simulink model "Ext_MFTyre_MFSwift_2sf"  (R2016b)
settings: Solver=ode4  StartTime=0.0  StopTime=20  FixedStep=0.0005  RelTol=1e-3
libraries: simulink_extras x16, mfswift_library x4, Solver_SF x2
settings Model: Creator=ywata  LastModifiedBy=mkhan
settings SolverCC: AutoInsertRateTranBlk=on
settings DataIOCC: ReturnWorkspaceOutputs=on
settings OptimizationCC: LifeSpan=inf
settings SFSimCC: SimUseLocalCustomCode=on
settings RTWCC: RTWUseLocalCustomCode=on

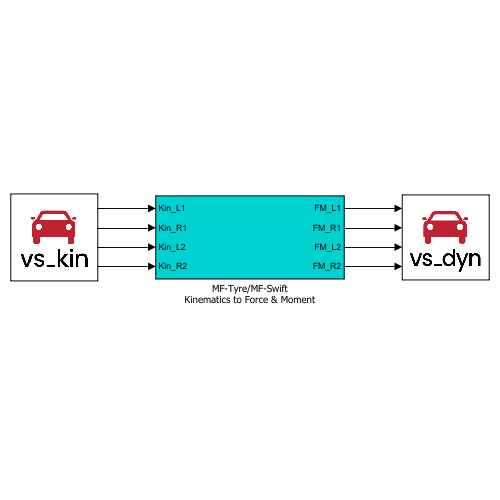
[thumbnail: Simulink's stored preview of the top-level diagram]
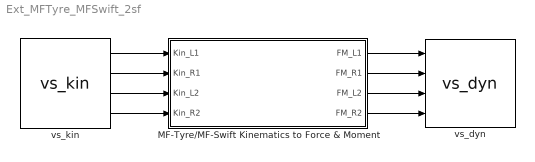
== system Ext_MFTyre_MFSwift_2sf ==
  MF-Tyre/MF-Swift Kinematics to Force & Moment : Subsystem
  vs_dyn : Solver_SF/CarSim Multi-Wrappers/vs_dyn  Priority=4  SIMFILE=simfile.sim
  vs_kin : Solver_SF/CarSim Multi-Wrappers/vs_kin  Priority=3  SIMFILE=simfile.sim
  wires:
  vs_kin/3 -> MF-Tyre/MF-Swift Kinematics to Force & Moment/3(Kin_L2)
  vs_kin/1 -> MF-Tyre/MF-Swift Kinematics to Force & Moment/1(Kin_L1)
  MF-Tyre/MF-Swift Kinematics to Force & Moment/1(FM_L1) -> vs_dyn/1
  MF-Tyre/MF-Swift Kinematics to Force & Moment/3(FM_L2) -> vs_dyn/3
  MF-Tyre/MF-Swift Kinematics to Force & Moment/2(FM_R1) -> vs_dyn/2
  MF-Tyre/MF-Swift Kinematics to Force & Moment/4(FM_R2) -> vs_dyn/4
  vs_kin/2 -> MF-Tyre/MF-Swift Kinematics to Force & Moment/2(Kin_R1)
  vs_kin/4 -> MF-Tyre/MF-Swift Kinematics to Force & Moment/4(Kin_R2)

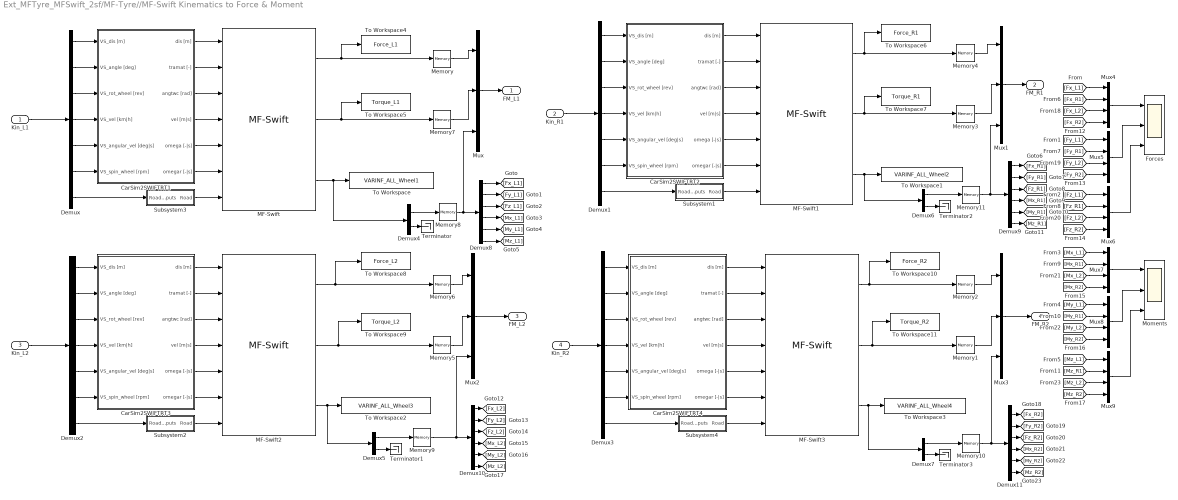
== system Ext_MFTyre_MFSwift_2sf/MF-Tyre//MF-Swift Kinematics to Force & Moment ==
  Kin_L1 : Inport
  Kin_R1 : Inport  Port=2
  Kin_L2 : Inport  Port=3
  Kin_R2 : Inport  Port=4
  CarSim2SWIFTRT1 : Subsystem
  CarSim2SWIFTRT2 : Subsystem
  CarSim2SWIFTRT3 : Subsystem
  CarSim2SWIFTRT4 : Subsystem
  Demux{,1..3} (4 alike) : Demux  Outputs=[3 3 1 3 3 1 3]
  Demux{8..11} (4 alike) : Demux  Outputs=6
  Demux4 : Demux  Outputs=[6 54]
  Demux5 : Demux  Outputs=[6 54]
  Demux6 : Demux  Outputs=[6,54]
  Demux7 : Demux  Outputs=[6 54]
  Forces : Scope  NumInputPorts=3
  MF-Swift : mfswift_library/MF-Swift  idtyre=1  tpfname='CS_car225_60R18.tir'  rdfname=''  road_mode=(3xxxx) external  side_mode=(x3xxx) symmetric  cnt_mode=(xx1xx) smooth road  dyn_mode=(xxx1x) relaxation behaviour  mf_mode=(xxxx4) combined  tv_model=Disabled  overwrite=off  use_mode=1e8  internal_solver=off  enable_rr_init=on  disp_debug=off
  MF-Swift1 : mfswift_library/MF-Swift  idtyre=2  tpfname='CS_car225_60R18.tir'  rdfname=''  road_mode=(3xxxx) external  side_mode=(x3xxx) symmetric  cnt_mode=(xx1xx) smooth road  dyn_mode=(xxx1x) relaxation behaviour  mf_mode=(xxxx4) combined  tv_model=Disabled  overwrite=off  use_mode=1e8  internal_solver=off  enable_rr_init=on  disp_debug=off
  MF-Swift2 : mfswift_library/MF-Swift  idtyre=3  tpfname='CS_car225_60R18.tir'  rdfname=''  road_mode=(3xxxx) external  side_mode=(x3xxx) symmetric  cnt_mode=(xx1xx) smooth road  dyn_mode=(xxx1x) relaxation behaviour  mf_mode=(xxxx4) combined  tv_model=Disabled  overwrite=off  use_mode=1e8  internal_solver=off  enable_rr_init=on  disp_debug=off
  MF-Swift3 : mfswift_library/MF-Swift  idtyre=4  tpfname='CS_car225_60R18.tir'  rdfname=''  road_mode=(3xxxx) external  side_mode=(x3xxx) symmetric  cnt_mode=(xx1xx) smooth road  dyn_mode=(xxx1x) relaxation behaviour  mf_mode=(xxxx4) combined  tv_model=Disabled  overwrite=off  use_mode=1e8  internal_solver=off  enable_rr_init=on  disp_debug=off
  Memory{,1..11} (12 alike) : Memory
  Moments : Scope  NumInputPorts=3
  Mux{,1..3} (4 alike) : Mux  Inputs=[3 3 6]
  Mux{4..9} (6 alike) : Mux
  Subsystem1 : Subsystem
  Subsystem2 : Subsystem
  Subsystem3 : Subsystem
  Subsystem4 : Subsystem
  Terminator{,1..3} (4 alike) : Terminator
  To Workspace : ToWorkspace  VariableName=VARINF_ALL_Wheel1  SampleTime=-1
  To Workspace1 : ToWorkspace  VariableName=VARINF_ALL_Wheel2  SampleTime=-1
  To Workspace10 : ToWorkspace  VariableName=Force_R2  SampleTime=-1
  To Workspace11 : ToWorkspace  VariableName=Torque_R2  SampleTime=-1
  To Workspace2 : ToWorkspace  VariableName=VARINF_ALL_Wheel3  SampleTime=-1
  To Workspace3 : ToWorkspace  VariableName=VARINF_ALL_Wheel4  SampleTime=-1
  To Workspace4 : ToWorkspace  VariableName=Force_L1  SampleTime=-1
  To Workspace5 : ToWorkspace  VariableName=Torque_L1  SampleTime=-1
  To Workspace6 : ToWorkspace  VariableName=Force_R1  SampleTime=-1
  To Workspace7 : ToWorkspace  VariableName=Torque_R1  SampleTime=-1
  To Workspace8 : ToWorkspace  VariableName=Force_L2  SampleTime=-1
  To Workspace9 : ToWorkspace  VariableName=Torque_L2  SampleTime=-1
  FM_L1 : Outport
  FM_R1 : Outport  Port=2
  FM_L2 : Outport  Port=3
  FM_R2 : Outport  Port=4
  wires:
  Mux/1 -> FM_L1/1
  Kin_L1/1 -> Demux/1
  MF-Swift1/1 -> Memory4/1, To Workspace6/1
  MF-Swift1/3 -> Demux6/1, To Workspace1/1
  CarSim2SWIFTRT2/1(dis [m]) -> MF-Swift1/1
  CarSim2SWIFTRT2/2(tramat [-]) -> MF-Swift1/2
  CarSim2SWIFTRT2/4(vel [m|s]) -> MF-Swift1/4
  CarSim2SWIFTRT2/5(omega [-|s]) -> MF-Swift1/5
  CarSim2SWIFTRT2/6(omegar [-|s]) -> MF-Swift1/6
  Mux1/1 -> FM_R1/1
  CarSim2SWIFTRT2/3(angtwc [rad]) -> MF-Swift1/3
  MF-Swift2/3 -> Demux5/1, To Workspace2/1
  CarSim2SWIFTRT3/1(dis [m]) -> MF-Swift2/1
  CarSim2SWIFTRT3/2(tramat [-]) -> MF-Swift2/2
  CarSim2SWIFTRT3/3(angtwc [rad]) -> MF-Swift2/3
  CarSim2SWIFTRT3/4(vel [m|s]) -> MF-Swift2/4
  CarSim2SWIFTRT3/5(omega [-|s]) -> MF-Swift2/5
  CarSim2SWIFTRT3/6(omegar [-|s]) -> MF-Swift2/6
  Mux2/1 -> FM_L2/1
  MF-Swift3/3 -> Demux7/1, To Workspace3/1
  CarSim2SWIFTRT4/1(dis [m]) -> MF-Swift3/1
  CarSim2SWIFTRT4/2(tramat [-]) -> MF-Swift3/2
  CarSim2SWIFTRT4/3(angtwc [rad]) -> MF-Swift3/3
  CarSim2SWIFTRT4/4(vel [m|s]) -> MF-Swift3/4
  CarSim2SWIFTRT4/5(omega [-|s]) -> MF-Swift3/5
  CarSim2SWIFTRT4/6(omegar [-|s]) -> MF-Swift3/6
  Mux3/1 -> FM_R2/1
  MF-Swift/2 -> Memory7/1, To Workspace5/1
  MF-Swift2/2 -> Memory5/1, To Workspace9/1
  MF-Swift1/2 -> Memory3/1, To Workspace7/1
  MF-Swift3/2 -> Memory1/1, To Workspace11/1
  MF-Swift/1 -> Memory/1, To Workspace4/1
  MF-Swift2/1 -> Memory6/1, To Workspace8/1
  MF-Swift3/1 -> Memory2/1, To Workspace10/1
  Subsystem2/1(Road) -> MF-Swift2/7
  Subsystem1/1(Road) -> MF-Swift1/7
  Subsystem4/1(Road) -> MF-Swift3/7
  MF-Swift/3 -> Demux4/1, To Workspace/1
  CarSim2SWIFTRT1/1(dis [m]) -> MF-Swift/1
  CarSim2SWIFTRT1/2(tramat [-]) -> MF-Swift/2
  CarSim2SWIFTRT1/3(angtwc [rad]) -> MF-Swift/3
  CarSim2SWIFTRT1/4(vel [m|s]) -> MF-Swift/4
  CarSim2SWIFTRT1/5(omega [-|s]) -> MF-Swift/5
  CarSim2SWIFTRT1/6(omegar [-|s]) -> MF-Swift/6
  Subsystem3/1(Road) -> MF-Swift/7
  Memory/1 -> Mux/1
  Memory7/1 -> Mux/2
  Memory6/1 -> Mux2/1
  Memory5/1 -> Mux2/2
  Memory4/1 -> Mux1/1
  Memory3/1 -> Mux1/2
  Memory2/1 -> Mux3/1
  Memory1/1 -> Mux3/2
  Demux4/1 -> Memory8/1
  Memory8/1 -> Demux8/1, Mux/3
  Demux5/1 -> Memory9/1
  Demux7/1 -> Memory10/1
  Demux6/1 -> Memory11/1
  Demux4/2 -> Terminator/1
  Demux5/2 -> Terminator1/1
  Demux6/2 -> Terminator2/1
  Demux7/2 -> Terminator3/1
  Demux/6 -> CarSim2SWIFTRT1/6(VS_spin_wheel [rpm])
  Demux/5 -> CarSim2SWIFTRT1/5(VS_angular_vel [deg|s])
  Demux/4 -> CarSim2SWIFTRT1/4(VS_vel [km|h])
  Demux/3 -> CarSim2SWIFTRT1/3(VS_rot_wheel [rev])
  Demux/2 -> CarSim2SWIFTRT1/2(VS_angle [deg])
  Demux/1 -> CarSim2SWIFTRT1/1(VS_dis [m])
  Kin_L2/1 -> Demux2/1
  Demux2/6 -> CarSim2SWIFTRT3/6(VS_spin_wheel [rpm])
  Demux2/3 -> CarSim2SWIFTRT3/3(VS_rot_wheel [rev])
  Demux2/1 -> CarSim2SWIFTRT3/1(VS_dis [m])
  Demux2/2 -> CarSim2SWIFTRT3/2(VS_angle [deg])
  Demux2/5 -> CarSim2SWIFTRT3/5(VS_angular_vel [deg|s])
  Demux2/4 -> CarSim2SWIFTRT3/4(VS_vel [km|h])
  Kin_R1/1 -> Demux1/1
  Demux1/6 -> CarSim2SWIFTRT2/6(VS_spin_wheel [rpm])
  Demux1/3 -> CarSim2SWIFTRT2/3(VS_rot_wheel [rev])
  Demux1/1 -> CarSim2SWIFTRT2/1(VS_dis [m])
  Demux1/2 -> CarSim2SWIFTRT2/2(VS_angle [deg])
  Demux1/5 -> CarSim2SWIFTRT2/5(VS_angular_vel [deg|s])
  Demux1/4 -> CarSim2SWIFTRT2/4(VS_vel [km|h])
  Kin_R2/1 -> Demux3/1
  Demux3/6 -> CarSim2SWIFTRT4/6(VS_spin_wheel [rpm])
  Demux3/3 -> CarSim2SWIFTRT4/3(VS_rot_wheel [rev])
  Demux3/1 -> CarSim2SWIFTRT4/1(VS_dis [m])
  Demux3/2 -> CarSim2SWIFTRT4/2(VS_angle [deg])
  Demux3/5 -> CarSim2SWIFTRT4/5(VS_angular_vel [deg|s])
  Demux3/4 -> CarSim2SWIFTRT4/4(VS_vel [km|h])
  Demux8/1 -> [Fx_L1]
  Demux8/2 -> [Fy_L1]
  Demux8/3 -> [Fz_L1]
  Demux8/4 -> [Mx_L1]
  Demux8/5 -> [My_L1]
  Demux8/6 -> [Mz_L1]
  Memory11/1 -> Demux9/1, Mux1/3
  Demux9/1 -> [Fx_R1]
  Demux9/6 -> [Mz_R1]
  Demux9/4 -> [Mx_R1]
  Demux9/3 -> [Fz_R1]
  Demux9/5 -> [My_R1]
  Demux9/2 -> [Fy_R1]
  Memory9/1 -> Mux2/3, Demux10/1
  Demux10/1 -> [Fx_L2]
  Demux10/6 -> [Mz_L2]
  Demux10/4 -> [Mx_L2]
  Demux10/3 -> [Fz_L2]
  Demux10/5 -> [My_L2]
  Demux10/2 -> [Fy_L2]
  Memory10/1 -> Mux3/3, Demux11/1
  Demux11/1 -> [Fx_R2]
  Demux11/6 -> [Mz_R2]
  Demux11/4 -> [Mx_R2]
  Demux11/3 -> [Fz_R2]
  Demux11/5 -> [My_R2]
  Demux11/2 -> [Fy_R2]
  [Fx_L1] -> Mux4/1
  [Fx_L2] -> Mux4/3
  [Fx_R1] -> Mux4/2
  [Fx_R2] -> Mux4/4
  [Fy_L1] -> Mux5/1
  [Fy_R1] -> Mux5/2
  [Fy_L2] -> Mux5/3
  [Fy_R2] -> Mux5/4
  [Fz_L1] -> Mux6/1
  [Fz_R1] -> Mux6/2
  [Fz_L2] -> Mux6/3
  [Fz_R2] -> Mux6/4
  Mux4/1 -> Forces/1
  Mux5/1 -> Forces/2
  Mux6/1 -> Forces/3
  Mux9/1 -> Moments/3
  [My_R1] -> Mux8/2
  [Mx_L1] -> Mux7/1
  [My_R2] -> Mux8/4
  Mux8/1 -> Moments/2
  Mux7/1 -> Moments/1
  [Mx_L2] -> Mux7/3
  [My_L1] -> Mux8/1
  [Mz_R1] -> Mux9/2
  [Mx_R1] -> Mux7/2
  [Mx_R2] -> Mux7/4
  [Mz_R2] -> Mux9/4
  [My_L2] -> Mux8/3
  [Mz_L2] -> Mux9/3
  [Mz_L1] -> Mux9/1
  Demux/7 -> Subsystem3/1(Road imputs)
  Demux3/7 -> Subsystem4/1(Road imputs)
  Demux1/7 -> Subsystem1/1(Road imputs)
  Demux2/7 -> Subsystem2/1(Road imputs)

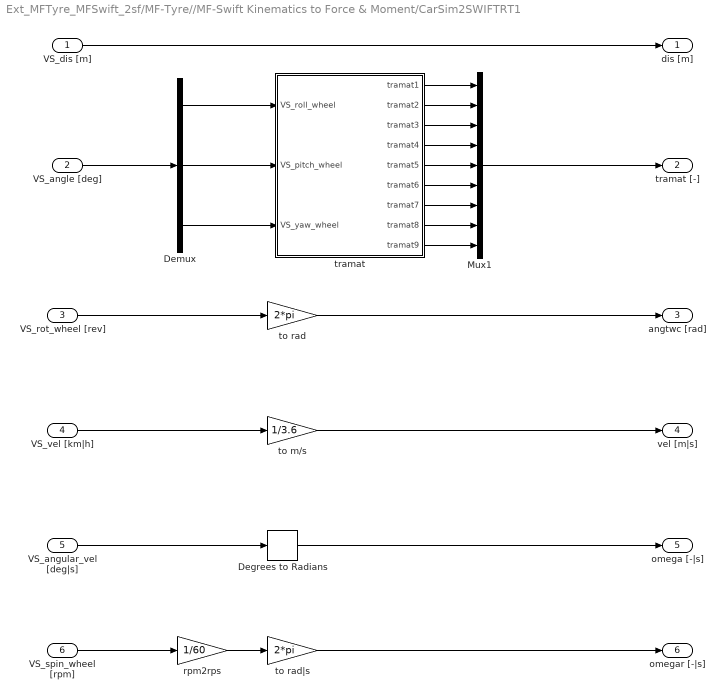
== system Ext_MFTyre_MFSwift_2sf/MF-Tyre//MF-Swift Kinematics to Force & Moment/CarSim2SWIFTRT1 ==
  VS_dis [m] : Inport
  VS_angle [deg] : Inport  Port=2
  VS_rot_wheel [rev] : Inport  Port=3
  VS_vel [km|h] : Inport  Port=4
  VS_angular_vel [deg|s] : Inport  Port=5
  VS_spin_wheel [rpm] : Inport  Port=6
  Degrees to Radians : simulink_extras/Transformations/Degrees to Radians
  Demux : Demux  Outputs=3
  Mux1 : Mux  Inputs=9
  rpm2rps : Gain  Gain=1/60
  to m/s : Gain  Gain=1/3.6
  to rad : Gain  Gain=2*pi
  to rad|s : Gain  Gain=2*pi
  tramat : Subsystem
  dis [m] : Outport
  tramat [-] : Outport  Port=2
  angtwc [rad] : Outport  Port=3
  vel [m|s] : Outport  Port=4
  omega [-|s] : Outport  Port=5
  omegar [-|s] : Outport  Port=6
  wires:
  Degrees to Radians/1 -> omega [-|s]/1
  to rad/1 -> angtwc [rad]/1
  tramat/1(tramat1) -> Mux1/1
  tramat/2(tramat2) -> Mux1/2
  tramat/3(tramat3) -> Mux1/3
  tramat/4(tramat4) -> Mux1/4
  tramat/5(tramat5) -> Mux1/5
  tramat/6(tramat6) -> Mux1/6
  tramat/7(tramat7) -> Mux1/7
  tramat/8(tramat8) -> Mux1/8
  tramat/9(tramat9) -> Mux1/9
  Mux1/1 -> tramat [-]/1
  VS_rot_wheel [rev]/1 -> to rad/1
  to m/s/1 -> vel [m|s]/1
  rpm2rps/1 -> to rad|s/1
  VS_spin_wheel [rpm]/1 -> rpm2rps/1
  to rad|s/1 -> omegar [-|s]/1
  VS_dis [m]/1 -> dis [m]/1
  VS_angle [deg]/1 -> Demux/1
  Demux/2 -> tramat/2(VS_pitch_wheel)
  Demux/1 -> tramat/1(VS_roll_wheel)
  Demux/3 -> tramat/3(VS_yaw_wheel)
  VS_vel [km|h]/1 -> to m/s/1
  VS_angular_vel [deg|s]/1 -> Degrees to Radians/1

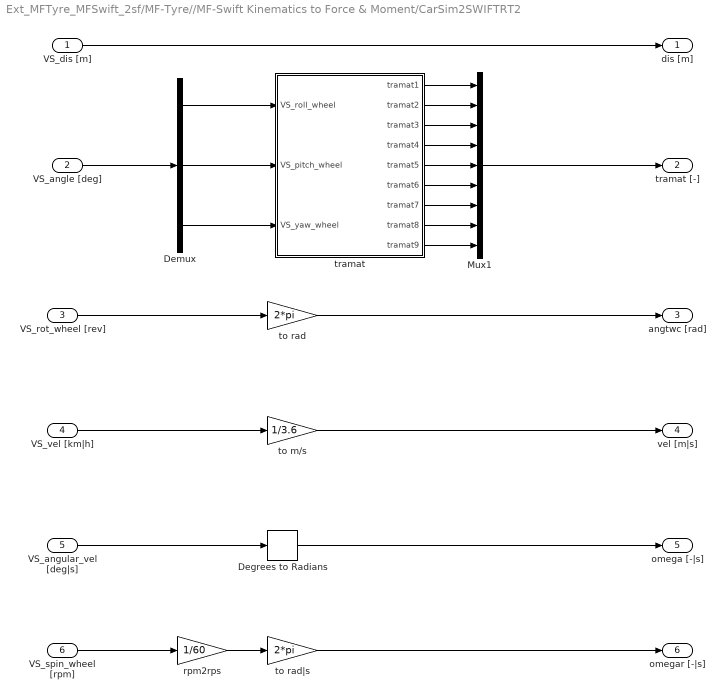
== system Ext_MFTyre_MFSwift_2sf/MF-Tyre//MF-Swift Kinematics to Force & Moment/CarSim2SWIFTRT2 ==
  VS_dis [m] : Inport
  VS_angle [deg] : Inport  Port=2
  VS_rot_wheel [rev] : Inport  Port=3
  VS_vel [km|h] : Inport  Port=4
  VS_angular_vel [deg|s] : Inport  Port=5
  VS_spin_wheel [rpm] : Inport  Port=6
  Degrees to Radians : simulink_extras/Transformations/Degrees to Radians
  Demux : Demux  Outputs=3
  Mux1 : Mux  Inputs=9
  rpm2rps : Gain  Gain=1/60
  to m/s : Gain  Gain=1/3.6
  to rad : Gain  Gain=2*pi
  to rad|s : Gain  Gain=2*pi
  tramat : Subsystem
  dis [m] : Outport
  tramat [-] : Outport  Port=2
  angtwc [rad] : Outport  Port=3
  vel [m|s] : Outport  Port=4
  omega [-|s] : Outport  Port=5
  omegar [-|s] : Outport  Port=6
  wires:
  Degrees to Radians/1 -> omega [-|s]/1
  to rad/1 -> angtwc [rad]/1
  tramat/1(tramat1) -> Mux1/1
  tramat/2(tramat2) -> Mux1/2
  tramat/3(tramat3) -> Mux1/3
  tramat/4(tramat4) -> Mux1/4
  tramat/5(tramat5) -> Mux1/5
  tramat/6(tramat6) -> Mux1/6
  tramat/7(tramat7) -> Mux1/7
  tramat/8(tramat8) -> Mux1/8
  tramat/9(tramat9) -> Mux1/9
  Mux1/1 -> tramat [-]/1
  VS_rot_wheel [rev]/1 -> to rad/1
  to m/s/1 -> vel [m|s]/1
  rpm2rps/1 -> to rad|s/1
  VS_spin_wheel [rpm]/1 -> rpm2rps/1
  to rad|s/1 -> omegar [-|s]/1
  VS_dis [m]/1 -> dis [m]/1
  VS_angle [deg]/1 -> Demux/1
  Demux/2 -> tramat/2(VS_pitch_wheel)
  Demux/1 -> tramat/1(VS_roll_wheel)
  Demux/3 -> tramat/3(VS_yaw_wheel)
  VS_vel [km|h]/1 -> to m/s/1
  VS_angular_vel [deg|s]/1 -> Degrees to Radians/1

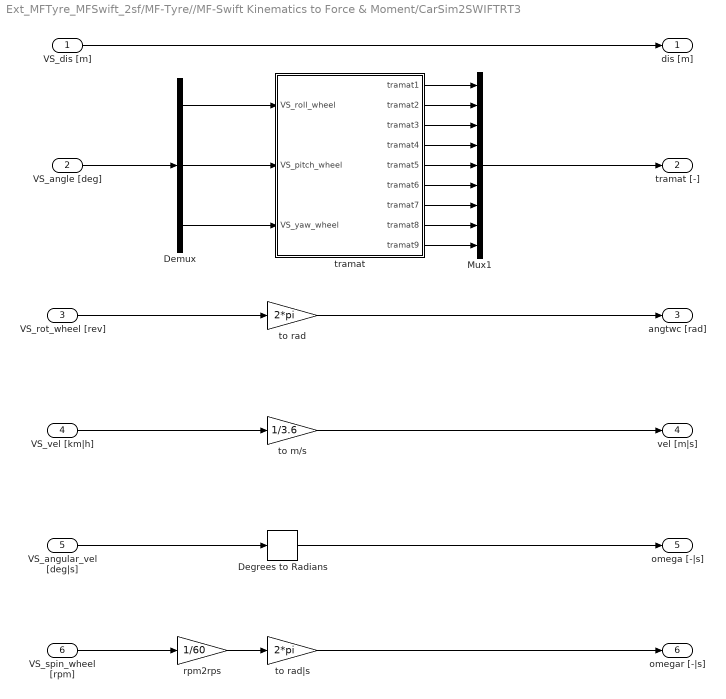
== system Ext_MFTyre_MFSwift_2sf/MF-Tyre//MF-Swift Kinematics to Force & Moment/CarSim2SWIFTRT3 ==
  VS_dis [m] : Inport
  VS_angle [deg] : Inport  Port=2
  VS_rot_wheel [rev] : Inport  Port=3
  VS_vel [km|h] : Inport  Port=4
  VS_angular_vel [deg|s] : Inport  Port=5
  VS_spin_wheel [rpm] : Inport  Port=6
  Degrees to Radians : simulink_extras/Transformations/Degrees to Radians
  Demux : Demux  Outputs=3
  Mux1 : Mux  Inputs=9
  rpm2rps : Gain  Gain=1/60
  to m/s : Gain  Gain=1/3.6
  to rad : Gain  Gain=2*pi
  to rad|s : Gain  Gain=2*pi
  tramat : Subsystem
  dis [m] : Outport
  tramat [-] : Outport  Port=2
  angtwc [rad] : Outport  Port=3
  vel [m|s] : Outport  Port=4
  omega [-|s] : Outport  Port=5
  omegar [-|s] : Outport  Port=6
  wires:
  Degrees to Radians/1 -> omega [-|s]/1
  to rad/1 -> angtwc [rad]/1
  tramat/1(tramat1) -> Mux1/1
  tramat/2(tramat2) -> Mux1/2
  tramat/3(tramat3) -> Mux1/3
  tramat/4(tramat4) -> Mux1/4
  tramat/5(tramat5) -> Mux1/5
  tramat/6(tramat6) -> Mux1/6
  tramat/7(tramat7) -> Mux1/7
  tramat/8(tramat8) -> Mux1/8
  tramat/9(tramat9) -> Mux1/9
  Mux1/1 -> tramat [-]/1
  VS_rot_wheel [rev]/1 -> to rad/1
  to m/s/1 -> vel [m|s]/1
  rpm2rps/1 -> to rad|s/1
  VS_spin_wheel [rpm]/1 -> rpm2rps/1
  to rad|s/1 -> omegar [-|s]/1
  VS_dis [m]/1 -> dis [m]/1
  VS_angle [deg]/1 -> Demux/1
  Demux/2 -> tramat/2(VS_pitch_wheel)
  Demux/1 -> tramat/1(VS_roll_wheel)
  Demux/3 -> tramat/3(VS_yaw_wheel)
  VS_vel [km|h]/1 -> to m/s/1
  VS_angular_vel [deg|s]/1 -> Degrees to Radians/1

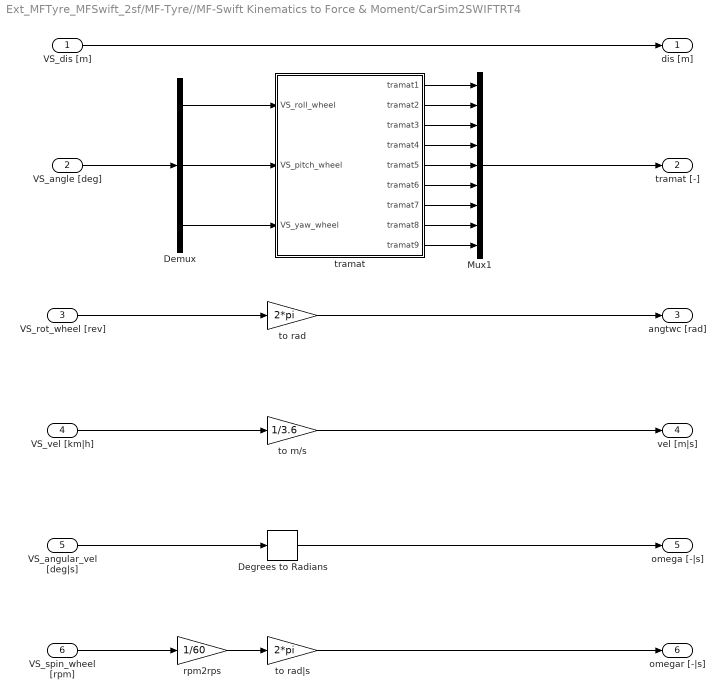
== system Ext_MFTyre_MFSwift_2sf/MF-Tyre//MF-Swift Kinematics to Force & Moment/CarSim2SWIFTRT4 ==
  VS_dis [m] : Inport
  VS_angle [deg] : Inport  Port=2
  VS_rot_wheel [rev] : Inport  Port=3
  VS_vel [km|h] : Inport  Port=4
  VS_angular_vel [deg|s] : Inport  Port=5
  VS_spin_wheel [rpm] : Inport  Port=6
  Degrees to Radians : simulink_extras/Transformations/Degrees to Radians
  Demux : Demux  Outputs=3
  Mux1 : Mux  Inputs=9
  rpm2rps : Gain  Gain=1/60
  to m/s : Gain  Gain=1/3.6
  to rad : Gain  Gain=2*pi
  to rad|s : Gain  Gain=2*pi
  tramat : Subsystem
  dis [m] : Outport
  tramat [-] : Outport  Port=2
  angtwc [rad] : Outport  Port=3
  vel [m|s] : Outport  Port=4
  omega [-|s] : Outport  Port=5
  omegar [-|s] : Outport  Port=6
  wires:
  Degrees to Radians/1 -> omega [-|s]/1
  to rad/1 -> angtwc [rad]/1
  tramat/1(tramat1) -> Mux1/1
  tramat/2(tramat2) -> Mux1/2
  tramat/3(tramat3) -> Mux1/3
  tramat/4(tramat4) -> Mux1/4
  tramat/5(tramat5) -> Mux1/5
  tramat/6(tramat6) -> Mux1/6
  tramat/7(tramat7) -> Mux1/7
  tramat/8(tramat8) -> Mux1/8
  tramat/9(tramat9) -> Mux1/9
  Mux1/1 -> tramat [-]/1
  VS_rot_wheel [rev]/1 -> to rad/1
  to m/s/1 -> vel [m|s]/1
  rpm2rps/1 -> to rad|s/1
  VS_spin_wheel [rpm]/1 -> rpm2rps/1
  to rad|s/1 -> omegar [-|s]/1
  VS_dis [m]/1 -> dis [m]/1
  VS_angle [deg]/1 -> Demux/1
  Demux/2 -> tramat/2(VS_pitch_wheel)
  Demux/1 -> tramat/1(VS_roll_wheel)
  Demux/3 -> tramat/3(VS_yaw_wheel)
  VS_vel [km|h]/1 -> to m/s/1
  VS_angular_vel [deg|s]/1 -> Degrees to Radians/1

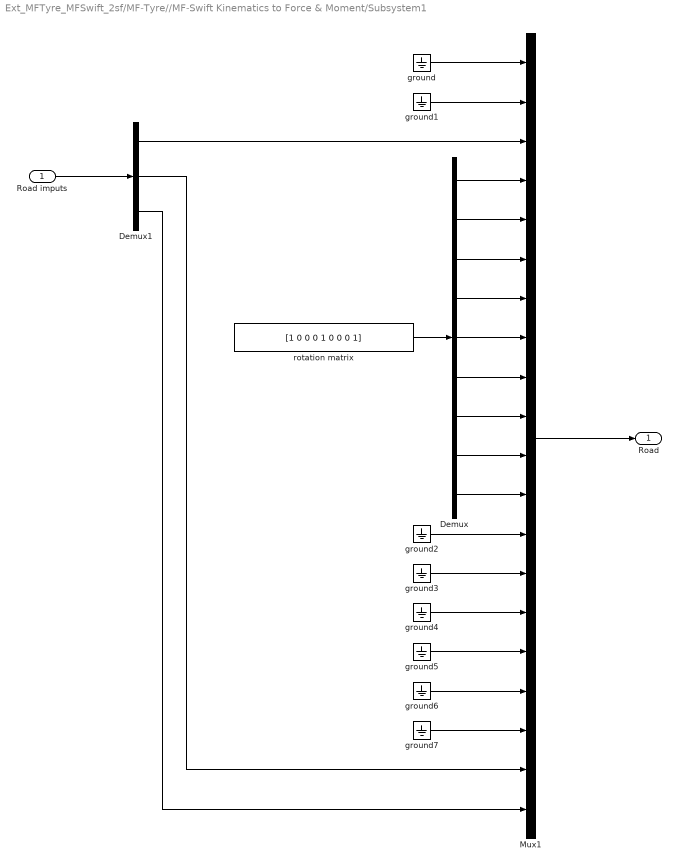
== system Ext_MFTyre_MFSwift_2sf/MF-Tyre//MF-Swift Kinematics to Force & Moment/Subsystem1 ==
  Road imputs : Inport
  Demux : Demux  Outputs=9
  Demux1 : Demux  Outputs=3
  Mux1 : Mux  Inputs=20
  ground{,1..7} (8 alike) : Ground
  rotation matrix : Constant  Value=[1 0 0 0 1 0 0 0 1]
  Road : Outport
  wires:
  Mux1/1 -> Road/1
  ground/1 -> Mux1/1
  ground1/1 -> Mux1/2
  ground2/1 -> Mux1/13
  ground3/1 -> Mux1/14
  ground4/1 -> Mux1/15
  ground5/1 -> Mux1/16
  ground6/1 -> Mux1/17
  ground7/1 -> Mux1/18
  Demux1/2 -> Mux1/19
  Demux1/3 -> Mux1/20
  rotation matrix/1 -> Demux/1
  Demux/1 -> Mux1/4
  Demux/2 -> Mux1/5
  Demux/3 -> Mux1/6
  Demux/4 -> Mux1/7
  Demux/5 -> Mux1/8
  Demux/6 -> Mux1/9
  Demux/7 -> Mux1/10
  Demux/8 -> Mux1/11
  Demux/9 -> Mux1/12
  Road imputs/1 -> Demux1/1
  Demux1/1 -> Mux1/3

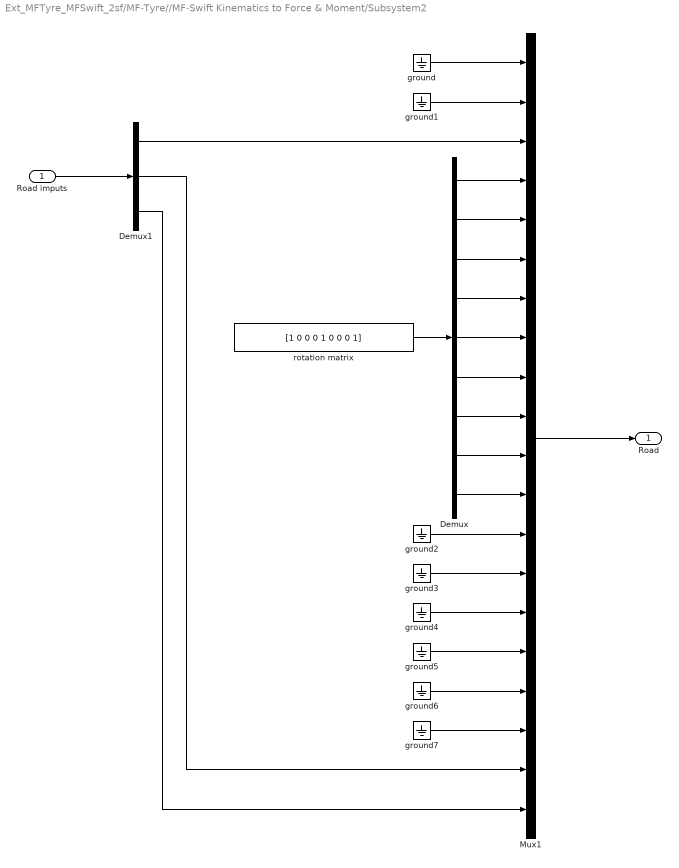
== system Ext_MFTyre_MFSwift_2sf/MF-Tyre//MF-Swift Kinematics to Force & Moment/Subsystem2 ==
  Road imputs : Inport
  Demux : Demux  Outputs=9
  Demux1 : Demux  Outputs=3
  Mux1 : Mux  Inputs=20
  ground{,1..7} (8 alike) : Ground
  rotation matrix : Constant  Value=[1 0 0 0 1 0 0 0 1]
  Road : Outport
  wires:
  Mux1/1 -> Road/1
  ground/1 -> Mux1/1
  ground1/1 -> Mux1/2
  ground2/1 -> Mux1/13
  ground3/1 -> Mux1/14
  ground4/1 -> Mux1/15
  ground5/1 -> Mux1/16
  ground6/1 -> Mux1/17
  ground7/1 -> Mux1/18
  Demux1/2 -> Mux1/19
  Demux1/3 -> Mux1/20
  rotation matrix/1 -> Demux/1
  Demux/1 -> Mux1/4
  Demux/2 -> Mux1/5
  Demux/3 -> Mux1/6
  Demux/4 -> Mux1/7
  Demux/5 -> Mux1/8
  Demux/6 -> Mux1/9
  Demux/7 -> Mux1/10
  Demux/8 -> Mux1/11
  Demux/9 -> Mux1/12
  Road imputs/1 -> Demux1/1
  Demux1/1 -> Mux1/3

== system Ext_MFTyre_MFSwift_2sf/MF-Tyre//MF-Swift Kinematics to Force & Moment/Subsystem3 ==
  Road imputs : Inport
  Demux : Demux  Outputs=9
  Demux1 : Demux  Outputs=3
  Mux1 : Mux  Inputs=20
  ground{,1..7} (8 alike) : Ground
  rotation matrix : Constant  Value=[1 0 0 0 1 0 0 0 1]
  Road : Outport
  wires:
  Mux1/1 -> Road/1
  ground/1 -> Mux1/1
  ground1/1 -> Mux1/2
  ground2/1 -> Mux1/13
  ground3/1 -> Mux1/14
  ground4/1 -> Mux1/15
  ground5/1 -> Mux1/16
  ground6/1 -> Mux1/17
  ground7/1 -> Mux1/18
  Demux1/2 -> Mux1/19
  Demux1/3 -> Mux1/20
  rotation matrix/1 -> Demux/1
  Demux/1 -> Mux1/4
  Demux/2 -> Mux1/5
  Demux/3 -> Mux1/6
  Demux/4 -> Mux1/7
  Demux/5 -> Mux1/8
  Demux/6 -> Mux1/9
  Demux/7 -> Mux1/10
  Demux/8 -> Mux1/11
  Demux/9 -> Mux1/12
  Road imputs/1 -> Demux1/1
  Demux1/1 -> Mux1/3

== system Ext_MFTyre_MFSwift_2sf/MF-Tyre//MF-Swift Kinematics to Force & Moment/Subsystem4 ==
  Road imputs : Inport
  Demux : Demux  Outputs=9
  Demux1 : Demux  Outputs=3
  Mux1 : Mux  Inputs=20
  ground{,1..7} (8 alike) : Ground
  rotation matrix : Constant  Value=[1 0 0 0 1 0 0 0 1]
  Road : Outport
  wires:
  Mux1/1 -> Road/1
  ground/1 -> Mux1/1
  ground1/1 -> Mux1/2
  ground2/1 -> Mux1/13
  ground3/1 -> Mux1/14
  ground4/1 -> Mux1/15
  ground5/1 -> Mux1/16
  ground6/1 -> Mux1/17
  ground7/1 -> Mux1/18
  Demux1/2 -> Mux1/19
  Demux1/3 -> Mux1/20
  rotation matrix/1 -> Demux/1
  Demux/1 -> Mux1/4
  Demux/2 -> Mux1/5
  Demux/3 -> Mux1/6
  Demux/4 -> Mux1/7
  Demux/5 -> Mux1/8
  Demux/6 -> Mux1/9
  Demux/7 -> Mux1/10
  Demux/8 -> Mux1/11
  Demux/9 -> Mux1/12
  Road imputs/1 -> Demux1/1
  Demux1/1 -> Mux1/3

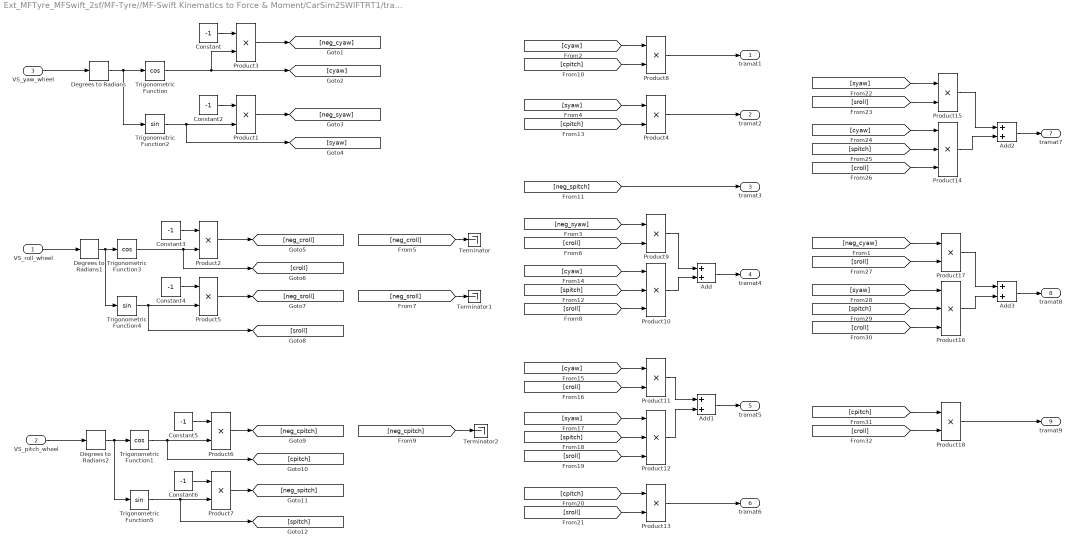
== system Ext_MFTyre_MFSwift_2sf/MF-Tyre//MF-Swift Kinematics to Force & Moment/CarSim2SWIFTRT1/tramat ==
  VS_roll_wheel : Inport
  VS_pitch_wheel : Inport  Port=2
  VS_yaw_wheel : Inport  Port=3
  Add{,1..3} (4 alike) : Sum
  Constant{,2..6} (6 alike) : Constant  Value=-1
  Degrees to Radians : simulink_extras/Transformations/Degrees to Radians
  Degrees to Radians1 : simulink_extras/Transformations/Degrees to Radians
  Degrees to Radians2 : simulink_extras/Transformations/Degrees to Radians
  Product{1..9,11,13,15,17..18} (14 alike) : Product  RndMeth=Zero
  Product{10,12,14,16} (4 alike) : Product  Inputs=3  RndMeth=Zero
  Terminator : Terminator
  Terminator1 : Terminator
  Terminator2 : Terminator
  Trigonometric Function : Trigonometry  Operator=cos
  Trigonometric Function1 : Trigonometry  Operator=cos
  Trigonometric Function2 : Trigonometry
  Trigonometric Function3 : Trigonometry  Operator=cos
  Trigonometric Function4 : Trigonometry
  Trigonometric Function5 : Trigonometry
  tramat1 : Outport
  tramat2 : Outport  Port=2
  tramat3 : Outport  Port=3
  tramat4 : Outport  Port=4
  tramat5 : Outport  Port=5
  tramat6 : Outport  Port=6
  tramat7 : Outport  Port=7
  tramat8 : Outport  Port=8
  tramat9 : Outport  Port=9
  wires:
  Constant/1 -> Product3/1
  Constant2/1 -> Product1/1
  Trigonometric Function2/1 -> Product1/2, [syaw]
  Constant3/1 -> Product2/1
  Trigonometric Function3/1 -> Product2/2, [croll]
  Constant4/1 -> Product5/1
  Trigonometric Function4/1 -> Product5/2, [sroll]
  Constant5/1 -> Product6/1
  Trigonometric Function1/1 -> Product6/2, [cpitch]
  Constant6/1 -> Product7/1
  Trigonometric Function5/1 -> Product7/2, [spitch]
  Product9/1 -> Add/1
  Product10/1 -> Add/2
  Add/1 -> tramat4/1
  Product3/1 -> [neg_cyaw]
  Trigonometric Function/1 -> Product3/2, [cyaw]
  Product1/1 -> [neg_syaw]
  Product2/1 -> [neg_croll]
  Product5/1 -> [neg_sroll]
  Product6/1 -> [neg_cpitch]
  Product7/1 -> [neg_spitch]
  [cyaw] -> Product8/1
  [cpitch] -> Product8/2
  Product8/1 -> tramat1/1
  [syaw] -> Product4/1
  [cpitch] -> Product4/2
  Product4/1 -> tramat2/1
  [neg_spitch] -> tramat3/1
  [neg_syaw] -> Product9/1
  [croll] -> Product9/2
  [cyaw] -> Product10/1
  [spitch] -> Product10/2
  [sroll] -> Product10/3
  [cyaw] -> Product11/1
  [croll] -> Product11/2
  [syaw] -> Product12/1
  [spitch] -> Product12/2
  [sroll] -> Product12/3
  Product11/1 -> Add1/1
  Product12/1 -> Add1/2
  Add1/1 -> tramat5/1
  [cpitch] -> Product13/1
  [sroll] -> Product13/2
  Product13/1 -> tramat6/1
  [syaw] -> Product15/1
  [sroll] -> Product15/2
  Product15/1 -> Add2/1
  [cyaw] -> Product14/1
  [spitch] -> Product14/2
  [croll] -> Product14/3
  Product14/1 -> Add2/2
  Add2/1 -> tramat7/1
  Add3/1 -> tramat8/1
  [neg_cyaw] -> Product17/1
  [sroll] -> Product17/2
  [syaw] -> Product16/1
  [spitch] -> Product16/2
  [croll] -> Product16/3
  Product17/1 -> Add3/1
  Product16/1 -> Add3/2
  [cpitch] -> Product18/1
  [croll] -> Product18/2
  Product18/1 -> tramat9/1
  [neg_croll] -> Terminator/1
  [neg_sroll] -> Terminator1/1
  [neg_cpitch] -> Terminator2/1
  Degrees to Radians/1 -> Trigonometric Function/1, Trigonometric Function2/1
  VS_roll_wheel/1 -> Degrees to Radians1/1
  Degrees to Radians1/1 -> Trigonometric Function3/1, Trigonometric Function4/1
  Degrees to Radians2/1 -> Trigonometric Function1/1, Trigonometric Function5/1
  VS_pitch_wheel/1 -> Degrees to Radians2/1
  VS_yaw_wheel/1 -> Degrees to Radians/1

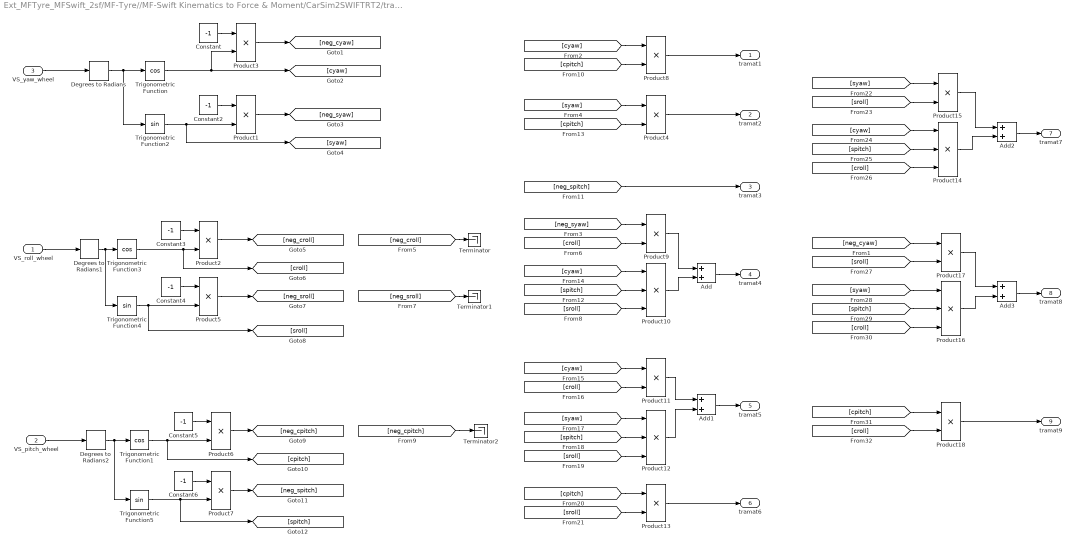
== system Ext_MFTyre_MFSwift_2sf/MF-Tyre//MF-Swift Kinematics to Force & Moment/CarSim2SWIFTRT2/tramat ==
  VS_roll_wheel : Inport
  VS_pitch_wheel : Inport  Port=2
  VS_yaw_wheel : Inport  Port=3
  Add{,1..3} (4 alike) : Sum
  Constant{,2..6} (6 alike) : Constant  Value=-1
  Degrees to Radians : simulink_extras/Transformations/Degrees to Radians
  Degrees to Radians1 : simulink_extras/Transformations/Degrees to Radians
  Degrees to Radians2 : simulink_extras/Transformations/Degrees to Radians
  Product{1..9,11,13,15,17..18} (14 alike) : Product  RndMeth=Zero
  Product{10,12,14,16} (4 alike) : Product  Inputs=3  RndMeth=Zero
  Terminator : Terminator
  Terminator1 : Terminator
  Terminator2 : Terminator
  Trigonometric Function : Trigonometry  Operator=cos
  Trigonometric Function1 : Trigonometry  Operator=cos
  Trigonometric Function2 : Trigonometry
  Trigonometric Function3 : Trigonometry  Operator=cos
  Trigonometric Function4 : Trigonometry
  Trigonometric Function5 : Trigonometry
  tramat1 : Outport
  tramat2 : Outport  Port=2
  tramat3 : Outport  Port=3
  tramat4 : Outport  Port=4
  tramat5 : Outport  Port=5
  tramat6 : Outport  Port=6
  tramat7 : Outport  Port=7
  tramat8 : Outport  Port=8
  tramat9 : Outport  Port=9
  wires:
  Constant/1 -> Product3/1
  Constant2/1 -> Product1/1
  Trigonometric Function2/1 -> Product1/2, [syaw]
  Constant3/1 -> Product2/1
  Trigonometric Function3/1 -> Product2/2, [croll]
  Constant4/1 -> Product5/1
  Trigonometric Function4/1 -> Product5/2, [sroll]
  Constant5/1 -> Product6/1
  Trigonometric Function1/1 -> Product6/2, [cpitch]
  Constant6/1 -> Product7/1
  Trigonometric Function5/1 -> Product7/2, [spitch]
  Product9/1 -> Add/1
  Product10/1 -> Add/2
  Add/1 -> tramat4/1
  Product3/1 -> [neg_cyaw]
  Trigonometric Function/1 -> Product3/2, [cyaw]
  Product1/1 -> [neg_syaw]
  Product2/1 -> [neg_croll]
  Product5/1 -> [neg_sroll]
  Product6/1 -> [neg_cpitch]
  Product7/1 -> [neg_spitch]
  [cyaw] -> Product8/1
  [cpitch] -> Product8/2
  Product8/1 -> tramat1/1
  [syaw] -> Product4/1
  [cpitch] -> Product4/2
  Product4/1 -> tramat2/1
  [neg_spitch] -> tramat3/1
  [neg_syaw] -> Product9/1
  [croll] -> Product9/2
  [cyaw] -> Product10/1
  [spitch] -> Product10/2
  [sroll] -> Product10/3
  [cyaw] -> Product11/1
  [croll] -> Product11/2
  [syaw] -> Product12/1
  [spitch] -> Product12/2
  [sroll] -> Product12/3
  Product11/1 -> Add1/1
  Product12/1 -> Add1/2
  Add1/1 -> tramat5/1
  [cpitch] -> Product13/1
  [sroll] -> Product13/2
  Product13/1 -> tramat6/1
  [syaw] -> Product15/1
  [sroll] -> Product15/2
  Product15/1 -> Add2/1
  [cyaw] -> Product14/1
  [spitch] -> Product14/2
  [croll] -> Product14/3
  Product14/1 -> Add2/2
  Add2/1 -> tramat7/1
  Add3/1 -> tramat8/1
  [neg_cyaw] -> Product17/1
  [sroll] -> Product17/2
  [syaw] -> Product16/1
  [spitch] -> Product16/2
  [croll] -> Product16/3
  Product17/1 -> Add3/1
  Product16/1 -> Add3/2
  [cpitch] -> Product18/1
  [croll] -> Product18/2
  Product18/1 -> tramat9/1
  [neg_croll] -> Terminator/1
  [neg_sroll] -> Terminator1/1
  [neg_cpitch] -> Terminator2/1
  Degrees to Radians/1 -> Trigonometric Function/1, Trigonometric Function2/1
  VS_roll_wheel/1 -> Degrees to Radians1/1
  Degrees to Radians1/1 -> Trigonometric Function3/1, Trigonometric Function4/1
  Degrees to Radians2/1 -> Trigonometric Function1/1, Trigonometric Function5/1
  VS_pitch_wheel/1 -> Degrees to Radians2/1
  VS_yaw_wheel/1 -> Degrees to Radians/1

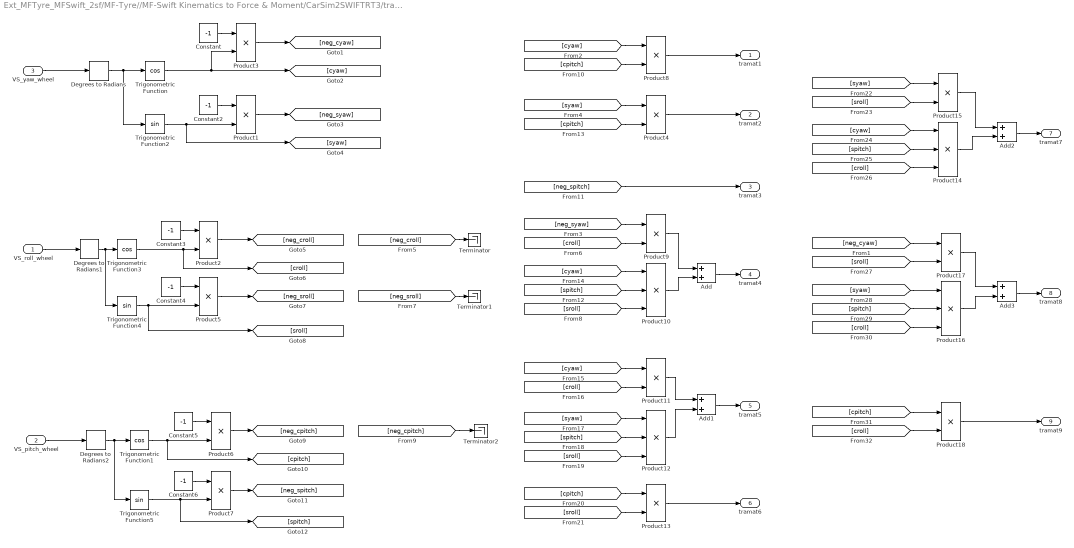
== system Ext_MFTyre_MFSwift_2sf/MF-Tyre//MF-Swift Kinematics to Force & Moment/CarSim2SWIFTRT3/tramat ==
  VS_roll_wheel : Inport
  VS_pitch_wheel : Inport  Port=2
  VS_yaw_wheel : Inport  Port=3
  Add{,1..3} (4 alike) : Sum
  Constant{,2..6} (6 alike) : Constant  Value=-1
  Degrees to Radians : simulink_extras/Transformations/Degrees to Radians
  Degrees to Radians1 : simulink_extras/Transformations/Degrees to Radians
  Degrees to Radians2 : simulink_extras/Transformations/Degrees to Radians
  Product{1..9,11,13,15,17..18} (14 alike) : Product  RndMeth=Zero
  Product{10,12,14,16} (4 alike) : Product  Inputs=3  RndMeth=Zero
  Terminator : Terminator
  Terminator1 : Terminator
  Terminator2 : Terminator
  Trigonometric Function : Trigonometry  Operator=cos
  Trigonometric Function1 : Trigonometry  Operator=cos
  Trigonometric Function2 : Trigonometry
  Trigonometric Function3 : Trigonometry  Operator=cos
  Trigonometric Function4 : Trigonometry
  Trigonometric Function5 : Trigonometry
  tramat1 : Outport
  tramat2 : Outport  Port=2
  tramat3 : Outport  Port=3
  tramat4 : Outport  Port=4
  tramat5 : Outport  Port=5
  tramat6 : Outport  Port=6
  tramat7 : Outport  Port=7
  tramat8 : Outport  Port=8
  tramat9 : Outport  Port=9
  wires:
  Constant/1 -> Product3/1
  Constant2/1 -> Product1/1
  Trigonometric Function2/1 -> Product1/2, [syaw]
  Constant3/1 -> Product2/1
  Trigonometric Function3/1 -> Product2/2, [croll]
  Constant4/1 -> Product5/1
  Trigonometric Function4/1 -> Product5/2, [sroll]
  Constant5/1 -> Product6/1
  Trigonometric Function1/1 -> Product6/2, [cpitch]
  Constant6/1 -> Product7/1
  Trigonometric Function5/1 -> Product7/2, [spitch]
  Product9/1 -> Add/1
  Product10/1 -> Add/2
  Add/1 -> tramat4/1
  Product3/1 -> [neg_cyaw]
  Trigonometric Function/1 -> Product3/2, [cyaw]
  Product1/1 -> [neg_syaw]
  Product2/1 -> [neg_croll]
  Product5/1 -> [neg_sroll]
  Product6/1 -> [neg_cpitch]
  Product7/1 -> [neg_spitch]
  [cyaw] -> Product8/1
  [cpitch] -> Product8/2
  Product8/1 -> tramat1/1
  [syaw] -> Product4/1
  [cpitch] -> Product4/2
  Product4/1 -> tramat2/1
  [neg_spitch] -> tramat3/1
  [neg_syaw] -> Product9/1
  [croll] -> Product9/2
  [cyaw] -> Product10/1
  [spitch] -> Product10/2
  [sroll] -> Product10/3
  [cyaw] -> Product11/1
  [croll] -> Product11/2
  [syaw] -> Product12/1
  [spitch] -> Product12/2
  [sroll] -> Product12/3
  Product11/1 -> Add1/1
  Product12/1 -> Add1/2
  Add1/1 -> tramat5/1
  [cpitch] -> Product13/1
  [sroll] -> Product13/2
  Product13/1 -> tramat6/1
  [syaw] -> Product15/1
  [sroll] -> Product15/2
  Product15/1 -> Add2/1
  [cyaw] -> Product14/1
  [spitch] -> Product14/2
  [croll] -> Product14/3
  Product14/1 -> Add2/2
  Add2/1 -> tramat7/1
  Add3/1 -> tramat8/1
  [neg_cyaw] -> Product17/1
  [sroll] -> Product17/2
  [syaw] -> Product16/1
  [spitch] -> Product16/2
  [croll] -> Product16/3
  Product17/1 -> Add3/1
  Product16/1 -> Add3/2
  [cpitch] -> Product18/1
  [croll] -> Product18/2
  Product18/1 -> tramat9/1
  [neg_croll] -> Terminator/1
  [neg_sroll] -> Terminator1/1
  [neg_cpitch] -> Terminator2/1
  Degrees to Radians/1 -> Trigonometric Function/1, Trigonometric Function2/1
  VS_roll_wheel/1 -> Degrees to Radians1/1
  Degrees to Radians1/1 -> Trigonometric Function3/1, Trigonometric Function4/1
  Degrees to Radians2/1 -> Trigonometric Function1/1, Trigonometric Function5/1
  VS_pitch_wheel/1 -> Degrees to Radians2/1
  VS_yaw_wheel/1 -> Degrees to Radians/1

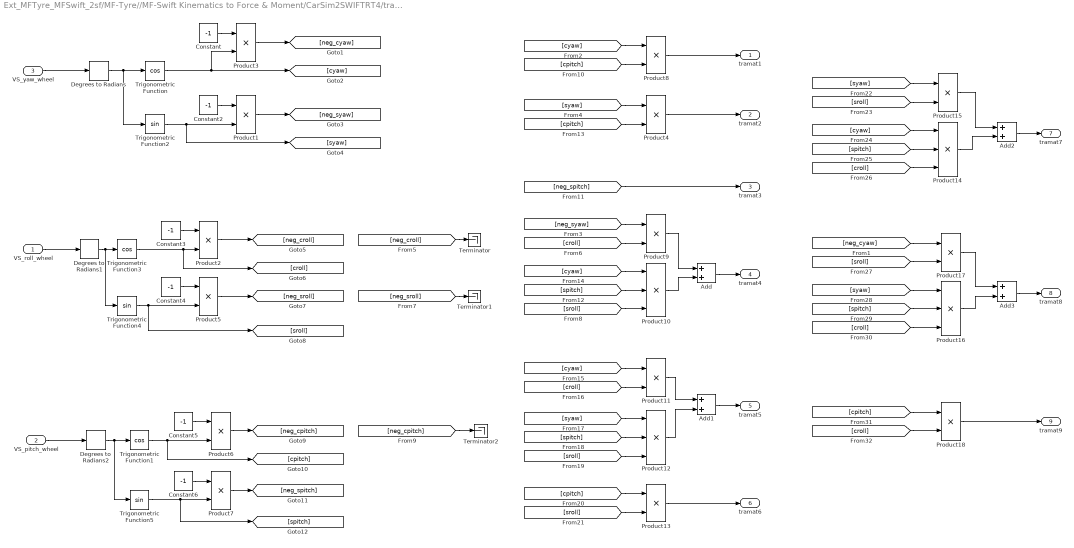
== system Ext_MFTyre_MFSwift_2sf/MF-Tyre//MF-Swift Kinematics to Force & Moment/CarSim2SWIFTRT4/tramat ==
  VS_roll_wheel : Inport
  VS_pitch_wheel : Inport  Port=2
  VS_yaw_wheel : Inport  Port=3
  Add{,1..3} (4 alike) : Sum
  Constant{,2..6} (6 alike) : Constant  Value=-1
  Degrees to Radians : simulink_extras/Transformations/Degrees to Radians
  Degrees to Radians1 : simulink_extras/Transformations/Degrees to Radians
  Degrees to Radians2 : simulink_extras/Transformations/Degrees to Radians
  Product{1..9,11,13,15,17..18} (14 alike) : Product  RndMeth=Zero
  Product{10,12,14,16} (4 alike) : Product  Inputs=3  RndMeth=Zero
  Terminator : Terminator
  Terminator1 : Terminator
  Terminator2 : Terminator
  Trigonometric Function : Trigonometry  Operator=cos
  Trigonometric Function1 : Trigonometry  Operator=cos
  Trigonometric Function2 : Trigonometry
  Trigonometric Function3 : Trigonometry  Operator=cos
  Trigonometric Function4 : Trigonometry
  Trigonometric Function5 : Trigonometry
  tramat1 : Outport
  tramat2 : Outport  Port=2
  tramat3 : Outport  Port=3
  tramat4 : Outport  Port=4
  tramat5 : Outport  Port=5
  tramat6 : Outport  Port=6
  tramat7 : Outport  Port=7
  tramat8 : Outport  Port=8
  tramat9 : Outport  Port=9
  wires:
  Constant/1 -> Product3/1
  Constant2/1 -> Product1/1
  Trigonometric Function2/1 -> Product1/2, [syaw]
  Constant3/1 -> Product2/1
  Trigonometric Function3/1 -> Product2/2, [croll]
  Constant4/1 -> Product5/1
  Trigonometric Function4/1 -> Product5/2, [sroll]
  Constant5/1 -> Product6/1
  Trigonometric Function1/1 -> Product6/2, [cpitch]
  Constant6/1 -> Product7/1
  Trigonometric Function5/1 -> Product7/2, [spitch]
  Product9/1 -> Add/1
  Product10/1 -> Add/2
  Add/1 -> tramat4/1
  Product3/1 -> [neg_cyaw]
  Trigonometric Function/1 -> Product3/2, [cyaw]
  Product1/1 -> [neg_syaw]
  Product2/1 -> [neg_croll]
  Product5/1 -> [neg_sroll]
  Product6/1 -> [neg_cpitch]
  Product7/1 -> [neg_spitch]
  [cyaw] -> Product8/1
  [cpitch] -> Product8/2
  Product8/1 -> tramat1/1
  [syaw] -> Product4/1
  [cpitch] -> Product4/2
  Product4/1 -> tramat2/1
  [neg_spitch] -> tramat3/1
  [neg_syaw] -> Product9/1
  [croll] -> Product9/2
  [cyaw] -> Product10/1
  [spitch] -> Product10/2
  [sroll] -> Product10/3
  [cyaw] -> Product11/1
  [croll] -> Product11/2
  [syaw] -> Product12/1
  [spitch] -> Product12/2
  [sroll] -> Product12/3
  Product11/1 -> Add1/1
  Product12/1 -> Add1/2
  Add1/1 -> tramat5/1
  [cpitch] -> Product13/1
  [sroll] -> Product13/2
  Product13/1 -> tramat6/1
  [syaw] -> Product15/1
  [sroll] -> Product15/2
  Product15/1 -> Add2/1
  [cyaw] -> Product14/1
  [spitch] -> Product14/2
  [croll] -> Product14/3
  Product14/1 -> Add2/2
  Add2/1 -> tramat7/1
  Add3/1 -> tramat8/1
  [neg_cyaw] -> Product17/1
  [sroll] -> Product17/2
  [syaw] -> Product16/1
  [spitch] -> Product16/2
  [croll] -> Product16/3
  Product17/1 -> Add3/1
  Product16/1 -> Add3/2
  [cpitch] -> Product18/1
  [croll] -> Product18/2
  Product18/1 -> tramat9/1
  [neg_croll] -> Terminator/1
  [neg_sroll] -> Terminator1/1
  [neg_cpitch] -> Terminator2/1
  Degrees to Radians/1 -> Trigonometric Function/1, Trigonometric Function2/1
  VS_roll_wheel/1 -> Degrees to Radians1/1
  Degrees to Radians1/1 -> Trigonometric Function3/1, Trigonometric Function4/1
  Degrees to Radians2/1 -> Trigonometric Function1/1, Trigonometric Function5/1
  VS_pitch_wheel/1 -> Degrees to Radians2/1
  VS_yaw_wheel/1 -> Degrees to Radians/1
